simulink model "simulation_basic"  (R2022b)
settings: Solver=ode4  StartTime=0.0  StopTime=10  FixedStep=5e-7  MaxStep=1e-6  RelTol=1e-3
undefined symbols (not defined in the file or in its folder): current, Down, inverter, motor, speed, Up
libraries: simulink x11, eeGeneralControl x7, mcbcontrolslib x5, slpidlib x3, SignalEditorBlockLib x2, spsTriangleGeneratorLib x2, spsSampleandHoldLib x1
(part 2 of 2)

== matlab function simulation_basic/MATLAB Function ==
  settings: updateMethod=DISCRETE
  data: v_alpha input; i_alpha_est output; v_beta input; i_alpha input; i_beta input; actual_rpm input; actual_theta input; Ts input; R input; L input; lambda_m input; i_beta_est output; i_d_est output; i_q_est output; omega_ele_est output; theta_ele_est output; omega_e_actual input; ekf_active output; rpm_thd input
function [i_alpha_est, i_beta_est, i_d_est, i_q_est, omega_ele_est, theta_ele_est, ekf_active] = ekf_observer(v_alpha, v_beta, i_alpha, i_beta, actual_rpm, actual_theta, Ts, R, L, lambda_m, omega_e_actual, rpm_thd)
persistent x P ekf_initialized
if isempty(ekf_initialized)
    x = zeros(4, 1);
    P = eye(4) * 0.01;
    ekf_initialized = false;
end

% ----------------------------------------------------
% TRIGGER CONDITION: Run EKF when Actual RPM >= rpm_thd
% ----------------------------------------------------
if abs(actual_rpm) >= rpm_thd
    % Turn-on edge: Latch actual states at startup
    if ~ekf_initialized
        x = [i_alpha; ...          % Measured alpha current
             i_beta; ...           % Measured beta current
             omega_e_actual; ...   % Actual electrical speed at turn-on
             actual_theta];        % Actual electrical angle at turn-on
         
        P = diag([0.01, 0.01, 1.0, 0.01]); 
        ekf_initialized = true;
    end
    
    % Q_cont: [i_alpha, i_beta, omega_e, theta_e]
    % High Q for speed/angle allows fast tracking during dynamics
    Q_cont = diag([1.0, 1.0, 800.0, 100.0]); %Q3 was 10000
    Q = Q_cont * Ts;
    
    % Low R_cov tells the filter to trust clean Simulink measurements
    R_cov = diag([1e-1, 1e-1]); %was 1e-4
    % ------------------------------
    
    x1 = x(1); x2 = x(2); x3 = x(3); x4 = x(4);
    
    % Continuous-time state derivatives f_c(x,u)
    f_c1 = -(R/L)*x1 + (lambda_m/L)*x3*sin(x4) + (1/L)*v_alpha;
    f_c2 = -(R/L)*x2 - (lambda_m/L)*x3*cos(x4) + (1/L)*v_beta;
    f_c3 = 0;
    f_c4 = x3;
    
    f_c = [f_c1; f_c2; f_c3; f_c4];
    
    % 1. Prediction Step (Euler Discretization)
    x_pred = x + f_c * Ts;
    
    % Continuous Jacobian A
    A = [ -R/L,    0,     (lambda_m/L)*sin(x4),  (lambda_m/L)*x3*cos(x4);
           0,   -R/L,    -(lambda_m/L)*cos(x4),  (lambda_m/L)*x3*sin(x4);
           0,    0,           0,                      0;
           0,    0,           1,                      0 ];
           
    % Discrete State Transition Matrix F = I + A*Ts
    F = eye(4) + A * Ts;
    P_pred = F * P * F' + Q;
    
    % 2. Correction Step
    H = [1, 0, 0, 0; 
         0, 1, 0, 0];
     
    y = [i_alpha; i_beta];
    innovation = y - H * x_pred;
    S = H * P_pred * H' + R_cov;
    K = (P_pred * H') / S;
    
    x = x_pred + K * innovation;
    P = (eye(4) - K * H) * P_pred;
    
    % Normalize estimated angle [0, 2*pi]
    x(4) = mod(x(4), 2*pi);
    
    % Forward Park Transformation (Alpha/Beta -> d/q)
    i_d_est =  x(1) * cos(x(4)) + x(2) * sin(x(4));
    i_q_est = -x(1) * sin(x(4)) + x(2) * cos(x(4));
        
    % Estimated outputs
    i_alpha_est   = x(1);
    i_beta_est    = x(2);
    omega_ele_est = x(3);
    theta_ele_est = x(4);
    ekf_active    = 1;
else
    % Below threshold: Keep EKF reset
    ekf_initialized = false;
    
    i_alpha_est   = 0;
    i_beta_est    = 0;
    i_d_est       = 0;
    i_q_est       = 0;
    omega_ele_est = 0;
    theta_ele_est = 0;
    ekf_active    = 0;
end
